simulink model "CruiseControl_TestGen_Harness_"  (R2018a)
settings: Solver=FixedStepDiscrete  StartTime=0.0  StopTime=2  FixedStep=0.1  RelTol=1e-3  EnableMultiTasking=on
undefined symbols (not defined in the file): sldvsubsys
libraries: simulink x8, sldvlib x6
settings Model: Creator=colosky  LastModifiedBy=colosky
settings DataIOCC: LimitDataPoints=on  SaveFormat=Array  SaveOutput=off  SaveTime=off
settings OptimizationCC: DefaultParameterBehavior=Inlined  InlineInvariantSignals=on  ExpressionDepthLimit=2147483647  InitFltsAndDblsToZero=on  NoFixptDivByZeroProtection=on  LifeSpan=inf
settings DebuggingCC: SignalInfNanChecking=warning  SaveWithParameterizedLinksMsg=none  UnderspecifiedInitializationDetection=Classic  MergeDetectMultiDrivingBlocksExec=none  SolverPrmCheckMsg=warning  FcnCallInpInsideContextMsg=warning  UniqueDataStoreMsg=warning  AllowSymbolicDim=off  StateNameClashWarn=warning  StrictBusMsg=ErrorOnBusTreatedAsVector  SFUnexpectedBacktrackingDiag=warning  SFNoUnconditionalDefaultTransitionDiag=warning  SFExecutionAtInitializationDiag=none
settings HardwareCC: ProdBitPerPointer=32  ProdBitPerSizeT=32  ProdBitPerPtrDiffT=32  ProdLargestAtomicFloat=None  ProdIntDivRoundTo=Undefined  ProdEndianess=Unspecified  ProdWordSize=32  ProdHWDeviceType=32-bit Generic
settings ModelReferenceCC: ModelReferenceNumInstancesAllowed=Single  PropagateSignalLabelsOutOfModel=off
settings SFSimCC: SimParseCustomCode=off  MATLABDynamicMemAlloc=off
settings RTWCC: SystemTargetFile=ert.tlc  TemplateMakefile=ert_default_tmf  GenerateReport=on  IncludeHyperlinkInReport=on  LaunchReport=on  PortableWordSizes=on  GenerateTraceInfo=on  GenerateTraceReport=on  GenerateTraceReportSl=on  GenerateTraceReportSf=on  GenerateTraceReportEml=on
settings CodeAppCC: IgnoreCustomStorageClasses=off  CustomSymbolStrGlobalVar=$N$M  StateflowObjectComments=on
settings ERTTargetCC: MultiwordLength=2048  GenerateSampleERTMain=on  InlinedParameterPlacement=NonHierarchical  ERTCustomFileTemplate=example_file_process.tlc  ConvertIfToSwitch=off  SuppressUnreachableDefaultCases=off
settings ConfigComp: CovEnable=on  CovScope=ReferencedModels  RecordCoverage=on  CovMetricSettings=dcme  CovModelRefEnable=Off  CovExternalEMLEnable=off  CovSFcnEnable=off  DVMode=DesignErrorDetection  DVMaxProcessTime=3000  DVDisplayUnsatisfiableObjectives=on  DVAutomaticStubbing=off  DVMakeOutputFilesUnique=off  DVModelCoverageObjectives=None  DVMaxTestCaseSteps=500  DVTestSuiteOptimization=IndividualObjectives  DVAssertions=EnableAll  DVProofAssumptions=EnableAll  DVCoverageDataFile=CruiseControlCovManual.cvt  DVDetectIntegerOverflow=off  DVDetectDeadLogic=on  DVDetectActiveLogic=on  DVDetectFloatOverflow=off  DVMaxViolationSteps=50  DVSaveExpectedOutput=on  DVSaveHarnessModel=on  DVHarnessModelFileName=$ModelName$_harness_SLDV  DVReportIncludeGraphics=on  DVDisplayResultsOnModel=on  PSAutoStubLUT=off

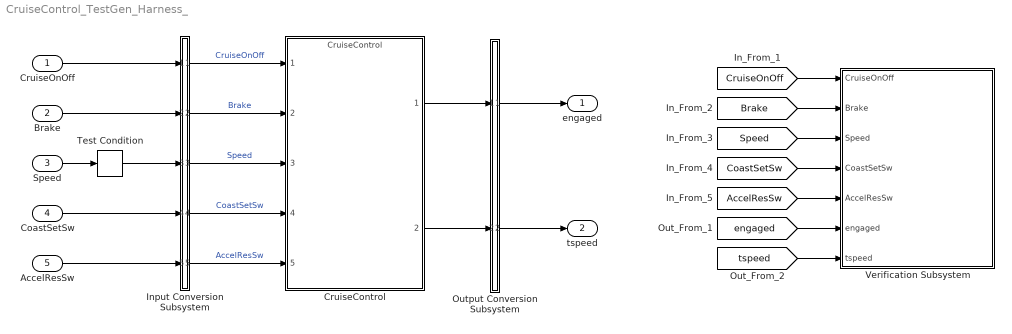
== system CruiseControl_TestGen_Harness_ ==
  CruiseOnOff : Inport  OutDataTypeStr=boolean  PortDimensions=[1]  SampleTime=0.1
  Brake : Inport  Port=2  OutDataTypeStr=boolean  PortDimensions=[1]  SampleTime=0.1
  Speed : Inport  Port=3  OutDataTypeStr=uint8  PortDimensions=[1]  SampleTime=0.1
  CoastSetSw : Inport  Port=4  OutDataTypeStr=boolean  PortDimensions=[1]  SampleTime=0.1
  AccelResSw : Inport  Port=5  OutDataTypeStr=boolean  PortDimensions=[1]  SampleTime=0.1
  CruiseControl : ModelReference  ModelNameDialog=CruiseControl  SimulationMode=Normal  ModelReferenceVersion=1.471
  Input Conversion Subsystem : Subsystem  Tag=__SLT_ICS__  Description=|
      | Signal spec.
      | and routing
      settings: AttributesFormatString=%<Description>
  Output Conversion Subsystem : Subsystem  Tag=__SLT_OCS__  Description=|
      | Signal spec.
      | and routing
      settings: AttributesFormatString=%<Description>
  Test Condition : sldvlib/Objectives and Constraints/Test Condition  enabled=on  customAVTBlockType=Test Condition  intervals=[20, 90]  initial=off  dispValues=on  outEnabled=on
      settings: AttributesFormatString=%<intervals>  SourceProductName=Simulink Design Verifier  SourceProductBaseCode=DV
  Verification Subsystem : Subsystem  Tag=VerificationSubsystem  DisableCoverage=on  LoadFcn=sldvsubsys('check')  TreatAsAtomicUnit=on  SimViewingDevice=on  mask(VerificationSubsystem){}
      mask init:
      | sldvsubsys('maskInit');
      settings: CopyFcn=sldvsubsys('copy');  OpenFcn=open_system(gcb,'force');
      settings: PreSaveFcn=|
      | set_param(gcb,'SimViewingDevice','on');
      | sldvsubsys('check');
      mask Help: helpview(fullfile(docroot,'toolbox','sldv','sldv.map'),'verificationsubsystem')
      mask Display: image(imread('sldvicon_versubsys.png','BackGroundColor',[1 1 1]),'center');
  engaged : Outport  OutDataTypeStr=boolean  PortDimensions=[1]
  tspeed : Outport  Port=2  OutDataTypeStr=uint8  PortDimensions=[1]
  wires:
  CruiseOnOff/1 -> Input Conversion Subsystem/1(Inport_1)
  Brake/1 -> Input Conversion Subsystem/2(Inport_2)
  Speed/1 -> Test Condition/1
  CoastSetSw/1 -> Input Conversion Subsystem/4(Inport_4)
  AccelResSw/1 -> Input Conversion Subsystem/5(Inport_5)
  Output Conversion Subsystem/1(Outport_1) -> engaged/1
  Output Conversion Subsystem/2(Outport_2) -> tspeed/1
  Input Conversion Subsystem/1(Outport_1) -> CruiseControl/1  "CruiseOnOff"
  Input Conversion Subsystem/2(Outport_2) -> CruiseControl/2  "Brake"
  Input Conversion Subsystem/3(Outport_3) -> CruiseControl/3  "Speed"
  Input Conversion Subsystem/4(Outport_4) -> CruiseControl/4  "CoastSetSw"
  Input Conversion Subsystem/5(Outport_5) -> CruiseControl/5  "AccelResSw"
  CruiseControl/1 -> Output Conversion Subsystem/1(Inport_1)
  CruiseControl/2 -> Output Conversion Subsystem/2(Inport_2)
  Test Condition/1 -> Input Conversion Subsystem/3(Inport_3)
  [CruiseOnOff] -> Verification Subsystem/1(CruiseOnOff)
  [Speed] -> Verification Subsystem/3(Speed)
  [AccelResSw] -> Verification Subsystem/5(AccelResSw)
  [engaged] -> Verification Subsystem/6(engaged)
  [Brake] -> Verification Subsystem/2(Brake)
  [tspeed] -> Verification Subsystem/7(tspeed)
  [CoastSetSw] -> Verification Subsystem/4(CoastSetSw)

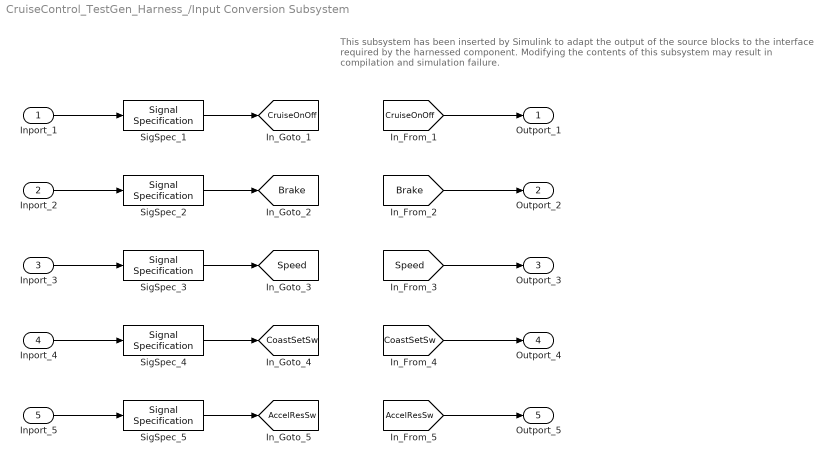
== system CruiseControl_TestGen_Harness_/Input Conversion Subsystem ==
  note: This subsystem has been inserted by Simulink to adapt the output of the source blocks to the interface required by the harnessed component.
      |  Modifying the contents of this subsystem may result in compilation and simulation failure.
  Inport_1 : Inport
  Inport_2 : Inport  Port=2
  Inport_3 : Inport  Port=3
  Inport_4 : Inport  Port=4
  Inport_5 : Inport  Port=5
  SigSpec_{1..2,4..5} (4 alike) : SignalSpecification  OutDataTypeStr=boolean  Dimensions=[1]  SampleTime=0.1
  SigSpec_3 : SignalSpecification  OutDataTypeStr=uint8  Dimensions=[1]  SampleTime=0.1
  Outport_1 : Outport
  Outport_2 : Outport  Port=2
  Outport_3 : Outport  Port=3
  Outport_4 : Outport  Port=4
  Outport_5 : Outport  Port=5
  tag scope: AccelResSw=global, Brake=global, CoastSetSw=global, CruiseOnOff=global, Speed=global
  wires:
  [CruiseOnOff] -> Outport_1/1
  SigSpec_1/1 -> [CruiseOnOff]
  Inport_1/1 -> SigSpec_1/1
  [Brake] -> Outport_2/1
  SigSpec_2/1 -> [Brake]
  Inport_2/1 -> SigSpec_2/1
  [Speed] -> Outport_3/1
  SigSpec_3/1 -> [Speed]
  Inport_3/1 -> SigSpec_3/1
  [CoastSetSw] -> Outport_4/1
  SigSpec_4/1 -> [CoastSetSw]
  Inport_4/1 -> SigSpec_4/1
  [AccelResSw] -> Outport_5/1
  SigSpec_5/1 -> [AccelResSw]
  Inport_5/1 -> SigSpec_5/1

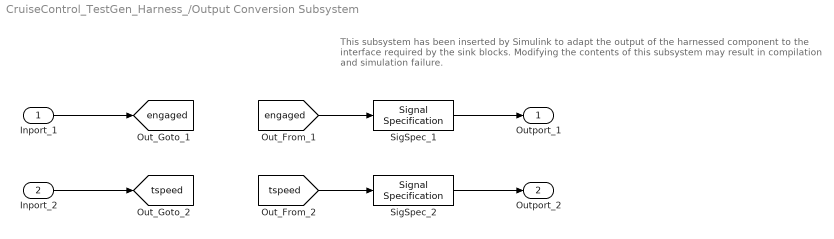
== system CruiseControl_TestGen_Harness_/Output Conversion Subsystem ==
  note: This subsystem has been inserted by Simulink to adapt the output of the harnessed component to the interface required by the sink blocks.
      |  Modifying the contents of this subsystem may result in compilation and simulation failure.
  Inport_1 : Inport
  Inport_2 : Inport  Port=2
  SigSpec_1 : SignalSpecification  OutDataTypeStr=boolean  Dimensions=[1]  SampleTime=0.1
  SigSpec_2 : SignalSpecification  OutDataTypeStr=uint8  Dimensions=[1]  SampleTime=0.1
  Outport_1 : Outport
  Outport_2 : Outport  Port=2
  tag scope: engaged=global, tspeed=global
  wires:
  Inport_1/1 -> [engaged]
  [engaged] -> SigSpec_1/1
  SigSpec_1/1 -> Outport_1/1
  Inport_2/1 -> [tspeed]
  [tspeed] -> SigSpec_2/1
  SigSpec_2/1 -> Outport_2/1

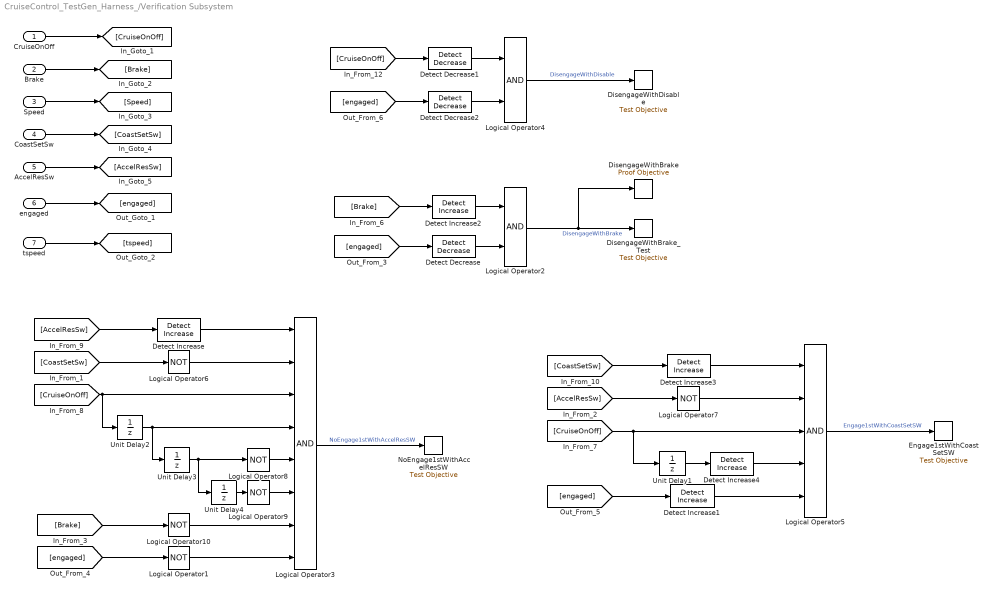
== system CruiseControl_TestGen_Harness_/Verification Subsystem ==
  CruiseOnOff : Inport  PortDimensions=1
  Brake : Inport  Port=2  PortDimensions=1
  Speed : Inport  Port=3  PortDimensions=1
  CoastSetSw : Inport  Port=4  PortDimensions=1
  AccelResSw : Inport  Port=5  PortDimensions=1
  engaged : Inport  Port=6  PortDimensions=1
  tspeed : Inport  Port=7  PortDimensions=1
  Detect Decrease : simulink/Logic and Bit Operations/Detect Decrease  vinit=false  OutDataTypeStr=boolean
  Detect Decrease1 : simulink/Logic and Bit Operations/Detect Decrease  vinit=false  OutDataTypeStr=boolean
  Detect Decrease2 : simulink/Logic and Bit Operations/Detect Decrease  vinit=false  OutDataTypeStr=boolean
  Detect Increase{,1,3..4} (4 alike) : simulink/Logic and Bit Operations/Detect Increase  vinit=0.0  OutDataTypeStr=boolean
  Detect Increase2 : simulink/Logic and Bit Operations/Detect Increase  vinit=false  OutDataTypeStr=boolean
  DisengageWithBrake : sldvlib/Objectives and Constraints/Proof Objective  enabled=on  customAVTBlockType=Proof Objective  intervals=true  dispValues=on  outEnabled=off  enableStopSim=off
      settings: AttributesFormatString=%<intervals>  SourceProductName=Simulink Design Verifier  SourceProductBaseCode=DV
  DisengageWithBrake_Test : sldvlib/Objectives and Constraints/Test Objective  enabled=on  customAVTBlockType=Test Objective  intervals=true  dispValues=on  outEnabled=off
      settings: AttributesFormatString=%<intervals>  SourceProductName=Simulink Design Verifier  SourceProductBaseCode=DV
  DisengageWithDisable : sldvlib/Objectives and Constraints/Test Objective  enabled=on  customAVTBlockType=Test Objective  intervals=true  dispValues=on  outEnabled=off
      settings: AttributesFormatString=%<intervals>  SourceProductName=Simulink Design Verifier  SourceProductBaseCode=DV
  Engage1stWithCoastSetSW : sldvlib/Objectives and Constraints/Test Objective  enabled=on  customAVTBlockType=Test Objective  intervals=true  dispValues=on  outEnabled=off
      settings: AttributesFormatString=%<intervals>  SourceProductName=Simulink Design Verifier  SourceProductBaseCode=DV
  Logical Operator{1,6..10} (6 alike) : Logic  Operator=NOT  AllPortsSameDT=off  OutDataTypeStr=boolean
  Logical Operator2 : Logic  AllPortsSameDT=off  OutDataTypeStr=boolean
  Logical Operator3 : Logic  Inputs=8  AllPortsSameDT=off  OutDataTypeStr=boolean
  Logical Operator4 : Logic  AllPortsSameDT=off  OutDataTypeStr=boolean
  Logical Operator5 : Logic  Inputs=5  AllPortsSameDT=off  OutDataTypeStr=boolean
  NoEngage1stWithAccelResSW : sldvlib/Objectives and Constraints/Test Objective  enabled=on  customAVTBlockType=Test Objective  intervals=true  dispValues=on  outEnabled=off
      settings: AttributesFormatString=%<intervals>  SourceProductName=Simulink Design Verifier  SourceProductBaseCode=DV
  Unit Delay1 : UnitDelay  InitialCondition=1  SampleTime=-1
  Unit Delay2 : UnitDelay  SampleTime=-1
  Unit Delay3 : UnitDelay  InitialCondition=1  SampleTime=-1
  Unit Delay4 : UnitDelay  InitialCondition=1  SampleTime=-1
  wires:
  Logical Operator6/1 -> Logical Operator3/2
  Detect Decrease2/1 -> Logical Operator4/2
  Logical Operator7/1 -> Logical Operator5/2
  Logical Operator9/1 -> Logical Operator3/6
  [engaged] -> Detect Increase1/1
  Detect Increase4/1 -> Logical Operator5/4
  [CoastSetSw] -> Detect Increase3/1
  Detect Increase3/1 -> Logical Operator5/1
  Unit Delay2/1 -> Unit Delay3/1, Logical Operator3/4
  Detect Decrease/1 -> Logical Operator2/2
  [CruiseOnOff] -> Detect Decrease1/1
  Logical Operator10/1 -> Logical Operator3/7
  [AccelResSw] -> Logical Operator7/1
  [CruiseOnOff] -> Logical Operator5/3, Unit Delay1/1
  [Brake] -> Detect Increase2/1
  Unit Delay4/1 -> Logical Operator9/1
  [CoastSetSw] -> Logical Operator6/1
  [CruiseOnOff] -> Logical Operator3/3, Unit Delay2/1
  Unit Delay3/1 -> Unit Delay4/1, Logical Operator8/1
  Logical Operator8/1 -> Logical Operator3/5
  [Brake] -> Logical Operator10/1
  Detect Increase1/1 -> Logical Operator5/5
  Unit Delay1/1 -> Detect Increase4/1
  [engaged] -> Detect Decrease2/1
  [AccelResSw] -> Detect Increase/1
  Detect Decrease1/1 -> Logical Operator4/1
  Detect Increase/1 -> Logical Operator3/1
  [engaged] -> Detect Decrease/1
  [engaged] -> Logical Operator1/1
  Logical Operator2/1 -> DisengageWithBrake/1, DisengageWithBrake_Test/1  "DisengageWithBrake"
  Logical Operator1/1 -> Logical Operator3/8
  Logical Operator5/1 -> Engage1stWithCoastSetSW/1  "Engage1stWithCoastSetSW"
  Detect Increase2/1 -> Logical Operator2/1
  Logical Operator3/1 -> NoEngage1stWithAccelResSW/1  "NoEngage1stWithAccelResSW"
  Logical Operator4/1 -> DisengageWithDisable/1  "DisengageWithDisable"
  CoastSetSw/1 -> [CoastSetSw]
  Speed/1 -> [Speed]
  CruiseOnOff/1 -> [CruiseOnOff]
  Brake/1 -> [Brake]
  AccelResSw/1 -> [AccelResSw]
  engaged/1 -> [engaged]
  tspeed/1 -> [tspeed]
